simulink model "inv_pend_R2011a"  (Simulink 9.1)
settings: Solver=ode45  StartTime=0.0  StopTime=10.0  RelTol=1e-3
InitFcn:
  | M = 0.5;
  | m = 0.2;
  | b = 0.1;
  | l = 0.3;
  | I = 0.006;
  | d_en = (M+m)*(I+m*l*l)-(m*l)*(m*l);
  | g = 9.8;
settings Model: SuppressorTable=22 serialization::archive 11 0 6 0 0 0 1 0  Creator=silveira  LastModifiedBy=silveira
settings DataIOCC: SaveFormat=StructureWithTime
settings DebuggingCC: AlgebraicLoopMsg=none  UnderspecifiedInitializationDetection=Simplified  MergeDetectMultiDrivingBlocksExec=error  FcnCallInpInsideContextMsg=warning  SFUnexpectedBacktrackingDiag=error  SFNoUnconditionalDefaultTransitionDiag=error
settings HardwareCC: ProdBitPerPointer=64  ProdLargestAtomicFloat=Float  ProdIntDivRoundTo=Zero  ProdEndianess=LittleEndian  ProdHWDeviceType=Specified
settings GRTTargetCC: TargetLangStandard=C99 (ISO)
settings ConfigComp: CovMetricSettings=dwe  CovHtmlReporting=off  CovSaveCumulativeToWorkspaceVar=off  CovSaveSingleToWorkspaceVar=off  CovExternalEMLEnable=on

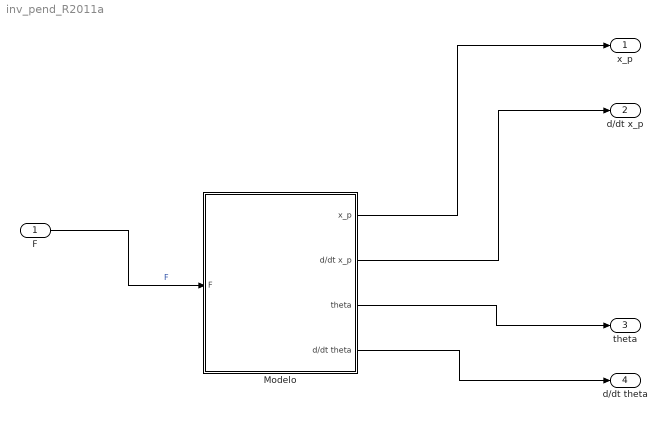
== system inv_pend_R2011a ==
  F : Inport
  Modelo : Subsystem
  x_p : Outport
  d/dt x_p : Outport  Port=2
  theta : Outport  Port=3
  d/dt theta : Outport  Port=4
  wires:
  F/1 -> Modelo/1(F)  "F"
  Modelo/1(x_p) -> x_p/1
  Modelo/2(d/dt x_p) -> d/dt x_p/1
  Modelo/3(theta) -> theta/1
  Modelo/4(d/dt theta) -> d/dt theta/1

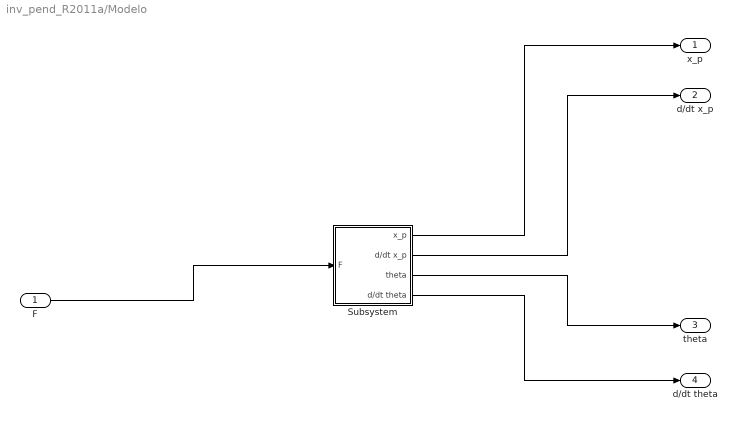
== system inv_pend_R2011a/Modelo ==
  F : Inport
  Subsystem : Subsystem
  x_p : Outport
  d/dt x_p : Outport  Port=2
  theta : Outport  Port=3
  d/dt theta : Outport  Port=4
  wires:
  F/1 -> Subsystem/1(F)
  Subsystem/1(x_p) -> x_p/1
  Subsystem/2(d/dt x_p) -> d/dt x_p/1
  Subsystem/3(theta) -> theta/1
  Subsystem/4(d/dt theta) -> d/dt theta/1

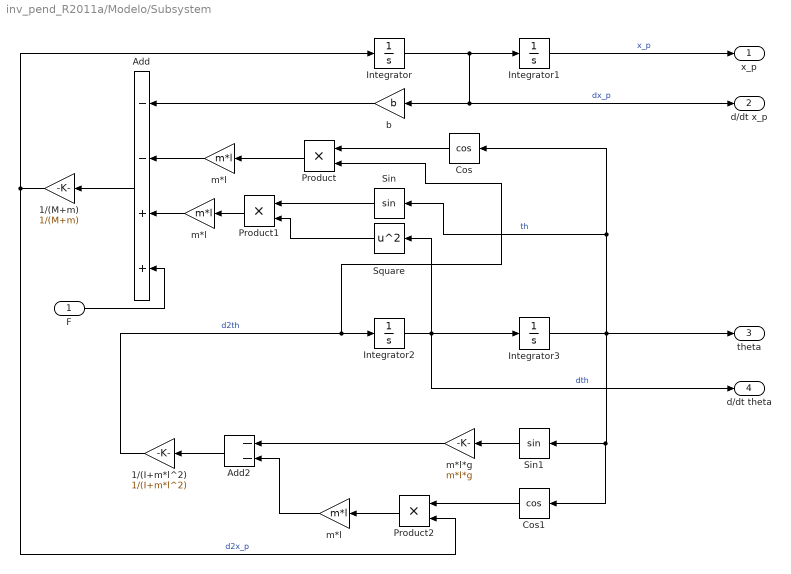
== system inv_pend_R2011a/Modelo/Subsystem ==
  F : Inport
  1/(I+m*l^2) : Gain  Gain=1/(I+m*l^2)
  1/(M+m) : Gain  Gain=1/(M+m)
  Add : Sum  Inputs=--++
  Add2 : Sum  Inputs=--
  Cos : Trigonometry  Operator=cos
  Cos1 : Trigonometry  Operator=cos  OutputSignalType=real
  Integrator : Integrator
  Integrator1 : Integrator
  Integrator2 : Integrator
  Integrator3 : Integrator  UpperSaturationLimit=pi+0.1  LowerSaturationLimit=pi-0.1
  Product : Product
  Product1 : Product
  Product2 : Product
  Sin : Trigonometry
  Sin1 : Trigonometry  OutputSignalType=real
  Square : Math  Operator=square  SaturateOnIntegerOverflow=on
  b : Gain  Gain=b
  m*l : Gain  Gain=m*l
  "m*l " : Gain  Gain=m*l
  "m*l  " : Gain  Gain=m*l
  m*l*g : Gain  Gain=m*l*g
  x_p : Outport
  d/dt x_p : Outport  Port=2
  theta : Outport  Port=3
  d/dt theta : Outport  Port=4
  wires:
  1/(I+m*l^2)/1 -> Product/2, Integrator2/1  "d2th"
  1/(M+m)/1 -> Product2/2, Integrator/1  "d2x_p"
  Integrator3/1 -> Cos1/1, Sin1/1, theta/1, Sin/1, Cos/1  "th"
  Add/1 -> 1/(M+m)/1
  Cos/1 -> Product/1
  Integrator1/1 -> x_p/1  "x_p"
  Integrator2/1 -> d/dt theta/1, Integrator3/1, Square/1  "dth"
  m*l*g/1 -> Add2/1
  Integrator/1 -> d/dt x_p/1, b/1, Integrator1/1  "dx_p"
  Cos1/1 -> Product2/1
  b/1 -> Add/1
  Sin/1 -> Product1/1
  Sin1/1 -> m*l*g/1
  Square/1 -> Product1/2
  F/1 -> Add/4
  Product1/1 -> "m*l "/1
  Product/1 -> m*l/1
  Add2/1 -> 1/(I+m*l^2)/1
  "m*l "/1 -> Add/3
  m*l/1 -> Add/2
  "m*l  "/1 -> Add2/2
  Product2/1 -> "m*l  "/1
